simulink model "p2_model"  (R2020a)
settings: Solver=VariableStepAuto  StartTime=0.0  StopTime=10  RelTol=1e-3
undefined symbols (not defined in the file): A, B, C, IC, L
settings Model: Creator=Tomo  LastModifiedBy=Tomo

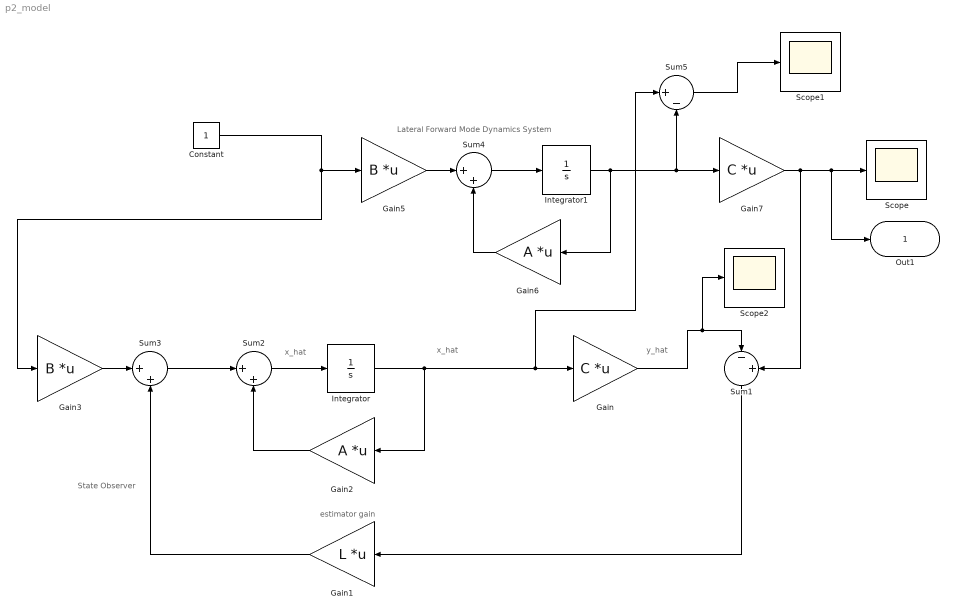
== system p2_model ==
  note: State Observer
  note: y_hat
  note: x_hat
  note: x_hat
  note: estimator gain
  note: Lateral Forward Mode Dynamics System
  Constant : Constant
  Gain : Gain  Gain=C  Multiplication=Matrix(K*u)
  Gain1 : Gain  Gain=L  Multiplication=Matrix(K*u)
  Gain2 : Gain  Gain=A  Multiplication=Matrix(K*u)
  Gain3 : Gain  Gain=B  Multiplication=Matrix(K*u)
  Gain5 : Gain  Gain=B  Multiplication=Matrix(K*u)
  Gain6 : Gain  Gain=A  Multiplication=Matrix(K*u)
  Gain7 : Gain  Gain=C  Multiplication=Matrix(K*u)
  Integrator : Integrator  InitialCondition=IC
  Integrator1 : Integrator  InitialCondition=IC
  Scope : Scope
  Scope1 : Scope
  Scope2 : Scope
  Sum1 : Sum  Inputs=|-+
  Sum2 : Sum  Inputs=|++
  Sum3 : Sum  Inputs=|++
  Sum4 : Sum  Inputs=|++
  Sum5 : Sum  Inputs=|+-
  Out1 : Outport
  wires:
  Constant/1 -> Gain3/1, Gain5/1
  Integrator1/1 -> Gain6/1, Sum5/2, Gain7/1
  Gain/1 -> Scope2/1, Sum1/1
  Sum1/1 -> Gain1/1
  Gain1/1 -> Sum3/2
  Gain2/1 -> Sum2/2
  Sum3/1 -> Sum2/1
  Sum2/1 -> Integrator/1
  Integrator/1 -> Gain2/1, Sum5/1, Gain/1
  Gain3/1 -> Sum3/1
  Gain5/1 -> Sum4/1
  Sum4/1 -> Integrator1/1
  Gain6/1 -> Sum4/2
  Gain7/1 -> Sum1/2, Out1/1, Scope/1
  Sum5/1 -> Scope1/1
